simulink model "PSCelec"  (R2020b)
settings: Solver=VariableStepAuto  StartTime=0.0  StopTime=100.0  RelTol=1e-3
undefined symbols (not defined in the file): sigbuilder_block
settings Model: Creator=colpari  LastModifiedBy=colpari

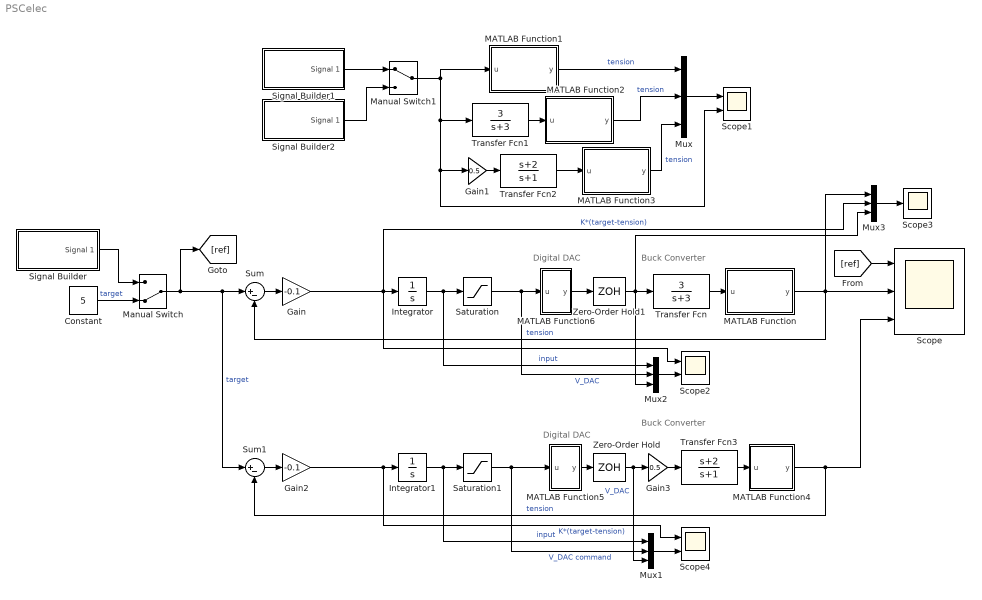
== system PSCelec ==
  note: Digital DAC
  note: Digital DAC
  note: Buck Converter
  note: Buck Converter
  Constant : Constant  Value=5
  Gain : Gain  Gain=-0.1
  Gain1 : Gain  Gain=0.5
  Gain2 : Gain  Gain=-0.1
  Gain3 : Gain  Gain=0.5
  Integrator : Integrator
  Integrator1 : Integrator
  MATLAB Function : MATLAB Function  TreatAsAtomicUnit=on
  MATLAB Function1 : MATLAB Function  TreatAsAtomicUnit=on
  MATLAB Function2 : MATLAB Function  TreatAsAtomicUnit=on
  MATLAB Function3 : MATLAB Function  TreatAsAtomicUnit=on
  MATLAB Function4 : MATLAB Function  TreatAsAtomicUnit=on
  MATLAB Function5 : MATLAB Function  TreatAsAtomicUnit=on
  MATLAB Function6 : MATLAB Function  TreatAsAtomicUnit=on
  Manual Switch : ManualSwitch  CurrentSetting=0
  Manual Switch1 : ManualSwitch
  Mux{,1..3} (4 alike) : Mux  Inputs=3
  Saturation : Saturate  UpperLimit=5  LowerLimit=1
  Saturation1 : Saturate  UpperLimit=5  LowerLimit=1
  Scope : Scope  NumInputPorts=3
  Scope1 : Scope  NumInputPorts=2
  Scope2 : Scope  NumInputPorts=2
  Scope3 : Scope
  Scope4 : Scope  NumInputPorts=2
  Signal Builder : Subsystem  Tag=STV Subsys  LoadFcn=sigbuilder_block('load');  StartFcn=sigbuilder_block('start');  StopFcn=sigbuilder_block('stop');  ClipboardFcn=sigbuilder_block('clipboard');  mask(Sigbuilder block){tuvar=[0:10]}
      mask help: Simulink:masks:SigbuilderBlock_MD
      mask init:
      | if ~strcmp(get_param(bdroot(gcbh),'SimulationStatus'),'stopped') tuvar = sigbuilder_block('maskInit'); end
      settings: CopyFcn=sigbuilder_block('copy');  DeleteFcn=sigbuilder_block('delete');  ModelCloseFcn=sigbuilder_block('modelClose');  PreSaveFcn=sigbuilder_block('preSave');  PauseFcn=sigbuilder_block('pause');  ContinueFcn=sigbuilder_block('continue');  NameChangeFcn=sigbuilder_block('namechange');  OpenFcn=sigbuilder_block('open',[337.5 87.75 550.5 399.75 ]);  CloseFcn=sigbuilder_block('close');
      mask Display: plot(0, 0, 100, 100,[2, 2, 32, 32, 2], [68, 8, 8, 68, 68],[32, 2], [38, 38], [32, 19, 2],[53, 60, 44], [32, 17, 17, 2],[16, 16, 31, 31]);txt = getActiveGroup(gcbh);text(2, 100, txt,'verticalAlignment', 'top');
  Signal Builder1 : Subsystem  Tag=STV Subsys  LoadFcn=sigbuilder_block('load');  StartFcn=sigbuilder_block('start');  StopFcn=sigbuilder_block('stop');  ClipboardFcn=sigbuilder_block('clipboard');  mask(Sigbuilder block){tuvar=[0:10]}
      mask help: Simulink:masks:SigbuilderBlock_MD
      mask init:
      | if ~strcmp(get_param(bdroot(gcbh),'SimulationStatus'),'stopped') tuvar = sigbuilder_block('maskInit'); end
      settings: CopyFcn=sigbuilder_block('copy');  DeleteFcn=sigbuilder_block('delete');  ModelCloseFcn=sigbuilder_block('modelClose');  PreSaveFcn=sigbuilder_block('preSave');  PauseFcn=sigbuilder_block('pause');  ContinueFcn=sigbuilder_block('continue');  NameChangeFcn=sigbuilder_block('namechange');  OpenFcn=sigbuilder_block('open',[437.6 199.2 550.4 400 ]);  CloseFcn=sigbuilder_block('close');
      mask Display: plot(0, 0, 100, 100,[2, 2, 32, 32, 2], [68, 8, 8, 68, 68],[32, 2], [38, 38], [32, 19, 2],[53, 60, 44], [32, 17, 17, 2],[16, 16, 31, 31]);txt = getActiveGroup(gcbh);text(2, 100, txt,'verticalAlignment', 'top');
  Signal Builder2 : Subsystem  Tag=STV Subsys  LoadFcn=sigbuilder_block('load');  StartFcn=sigbuilder_block('start');  StopFcn=sigbuilder_block('stop');  ClipboardFcn=sigbuilder_block('clipboard');  mask(Sigbuilder block){tuvar=[0:10]}
      mask help: Simulink:masks:SigbuilderBlock_MD
      mask init:
      | if ~strcmp(get_param(bdroot(gcbh),'SimulationStatus'),'stopped') tuvar = sigbuilder_block('maskInit'); end
      settings: CopyFcn=sigbuilder_block('copy');  DeleteFcn=sigbuilder_block('delete');  ModelCloseFcn=sigbuilder_block('modelClose');  PreSaveFcn=sigbuilder_block('preSave');  PauseFcn=sigbuilder_block('pause');  ContinueFcn=sigbuilder_block('continue');  NameChangeFcn=sigbuilder_block('namechange');  OpenFcn=sigbuilder_block('open',[337.5 87.75 550.5 399.75 ]);  CloseFcn=sigbuilder_block('close');
      mask Display: plot(0, 0, 100, 100,[2, 2, 32, 32, 2], [68, 8, 8, 68, 68],[32, 2], [38, 38], [32, 19, 2],[53, 60, 44], [32, 17, 17, 2],[16, 16, 31, 31]);txt = getActiveGroup(gcbh);text(2, 100, txt,'verticalAlignment', 'top');
  Sum : Sum  Inputs=|+-
  Sum1 : Sum  Inputs=|+-
  Transfer Fcn : TransferFcn  Numerator=[3]  Denominator=[1 3]
  Transfer Fcn1 : TransferFcn  Numerator=[3]  Denominator=[1 3]
  Transfer Fcn2 : TransferFcn  Numerator=[1 2]  Denominator=[1 1]
  Transfer Fcn3 : TransferFcn  Numerator=[1 2]  Denominator=[1 1]
  Zero-Order Hold : ZeroOrderHold  SampleTime=0.05
  Zero-Order Hold1 : ZeroOrderHold  SampleTime=0.05
  wires:
  MATLAB Function/1(y) -> Mux3/1, Scope/2, Sum/2  "tension"
  Sum/1 -> Gain/1
  Transfer Fcn/1 -> MATLAB Function/1(u)
  Signal Builder/1(Signal 1) -> Manual Switch/1
  MATLAB Function1/1(y) -> Mux/1  "tension"
  Manual Switch1/1 -> Scope1/2, Gain1/1, Transfer Fcn1/1, MATLAB Function1/1(u)
  Transfer Fcn1/1 -> MATLAB Function2/1(u)
  MATLAB Function2/1(y) -> Mux/2  "tension"
  Constant/1 -> Manual Switch/2  "target"
  Gain/1 -> Mux3/2, Scope2/1, Integrator/1  "K*(target-tension)"
  Saturation/1 -> Mux2/2, MATLAB Function6/1(u)  "V_DAC"
  Mux/1 -> Scope1/1
  Integrator/1 -> Mux2/1, Saturation/1  "input"
  Signal Builder1/1(Signal 1) -> Manual Switch1/1
  Signal Builder2/1(Signal 1) -> Manual Switch1/2
  Transfer Fcn2/1 -> MATLAB Function3/1(u)
  MATLAB Function3/1(y) -> Mux/3  "tension"
  Gain1/1 -> Transfer Fcn2/1
  MATLAB Function4/1(y) -> Scope/3, Sum1/2  "tension"
  Saturation1/1 -> MATLAB Function5/1(u), Mux1/2  "V_DAC command"
  Sum1/1 -> Gain2/1
  Gain2/1 -> Scope4/1, Integrator1/1  "K*(target-tension)"
  Integrator1/1 -> Mux1/1, Saturation1/1  "input"
  Transfer Fcn3/1 -> MATLAB Function4/1(u)
  Manual Switch/1 -> [ref], Sum1/1, Sum/1  "target"
  Gain3/1 -> Transfer Fcn3/1
  [ref] -> Scope/1
  MATLAB Function5/1(y) -> Zero-Order Hold/1
  Zero-Order Hold/1 -> Mux1/3, Gain3/1  "V_DAC"
  MATLAB Function6/1(y) -> Zero-Order Hold1/1
  Zero-Order Hold1/1 -> Mux3/3, Mux2/3, Transfer Fcn/1
  Mux1/1 -> Scope4/2
  Mux2/1 -> Scope2/2
  Mux3/1 -> Scope3/1

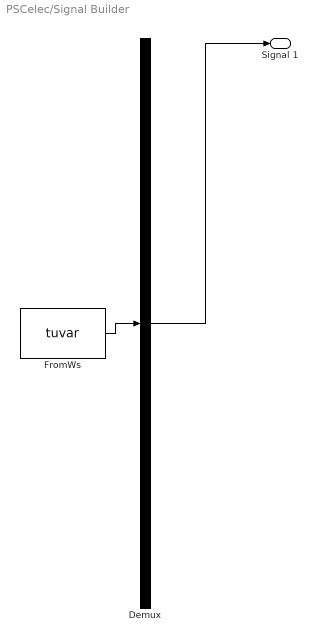
== system PSCelec/Signal Builder ==
  Demux : Demux  Tag=STV Demux  Outputs=1
      settings: DisplayOption=none
  FromWs : FromWorkspace  Tag=STV FromWs  VariableName=tuvar
      SigBuilderData=|
      | common.afterFinalStr = 'Extrapolate'
      | common.sampleTime = 0
      | dataSet.timeRange = [0 10]
      | dataSet.name = 'Group 1'
      | sbobj.Groups.Name = 'Group 1'
      | sbobj.Groups.Signals.Name = 'Signal 1'
      | sbobj.Groups.Signals.XData = [0 4 4 6 6 10]
      | sbobj.Groups.Signals.YData = [0 5 -0.02 1 0 0]
  Signal 1 : Outport  Tag=STV Outport
  wires:
  Demux/1 -> Signal 1/1
  FromWs/1 -> Demux/1

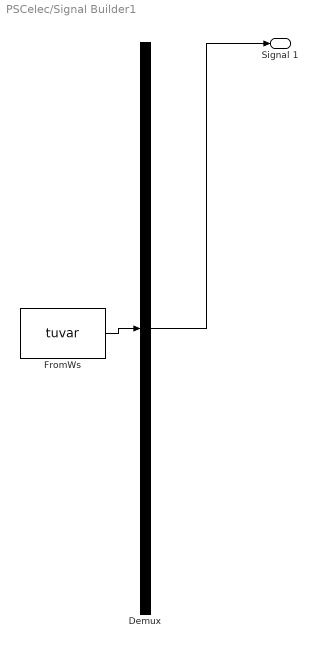
== system PSCelec/Signal Builder1 ==
  Demux : Demux  Tag=STV Demux  Outputs=1
      settings: DisplayOption=none
  FromWs : FromWorkspace  Tag=STV FromWs  VariableName=tuvar
      SigBuilderData=|
      | common.afterFinalStr = 'Extrapolate'
      | common.sampleTime = 0
      | dataSet.timeRange = [0 100]
      | dataSet.name = 'Group 1'
      | sbobj.Groups.Name = 'Group 1'
      | sbobj.Groups.Signals.Name = 'Signal 1'
      | sbobj.Groups.Signals.XData = [0 30 30 40 50 60 90 100]
      | sbobj.Groups.Signals.YData = [0 5 0 1 0 3 0 0]
      | sbobj.Groups.TimeRange = [0 100]
  Signal 1 : Outport  Tag=STV Outport
  wires:
  Demux/1 -> Signal 1/1
  FromWs/1 -> Demux/1

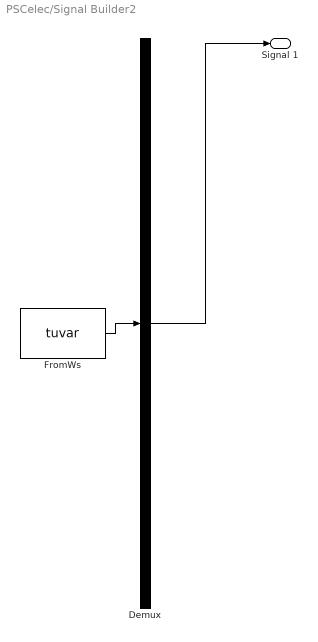
== system PSCelec/Signal Builder2 ==
  Demux : Demux  Tag=STV Demux  Outputs=1
      settings: DisplayOption=none
  FromWs : FromWorkspace  Tag=STV FromWs  VariableName=tuvar
      SigBuilderData=|
      | common.afterFinalStr = 'Extrapolate'
      | common.sampleTime = 0
      | dataSet.timeRange = [0 10]
      | dataSet.name = 'Group 1'
      | sbobj.Groups.Name = 'Group 1'
      | sbobj.Groups.Signals.Name = 'Signal 1'
      | sbobj.Groups.Signals.XData = [0 4 4 6 6 10]
      | sbobj.Groups.Signals.YData = [0 5 -0.02 1 0 0]
  Signal 1 : Outport  Tag=STV Outport
  wires:
  Demux/1 -> Signal 1/1
  FromWs/1 -> Demux/1

== matlab function PSCelec/MATLAB Function ==
  data: u input; y output
function y = fcn(u)

y = 16-2.9414*u;

== matlab function PSCelec/MATLAB Function2 ==
  data: u input; y output
function y = fcn(u)

y = 16-2.9414*u;

== matlab function PSCelec/MATLAB Function3 ==
  data: u input; y output
function y = fcn(u)

y = 16-2.9414*u;

== matlab function PSCelec/MATLAB Function4 ==
  data: u input; y output
function y = fcn(u)

y = 16-2.9414*u;

== matlab function PSCelec/MATLAB Function5 ==
  data: u input; y output
function y = fcn(u)
edges=0:1/4095:5;
y = discretize(u,edges)/4096;

== matlab function PSCelec/MATLAB Function6 ==
  data: u input; y output
function y = fcn(u)
edges=0:1/4095:5;
y = discretize(u,edges)/4096;

== matlab function PSCelec/MATLAB Function1 ==
  data: u input; y output
function y = fcn(u)

y = 16-2.9414*u;
